simulink model "simluation"  (R2015a)
settings: Solver=ode45  StartTime=0.0  StopTime=10.0  RelTol=1e-3
libraries: simulink x8
settings Model: Creator=Scott  LastModifiedBy=Scott

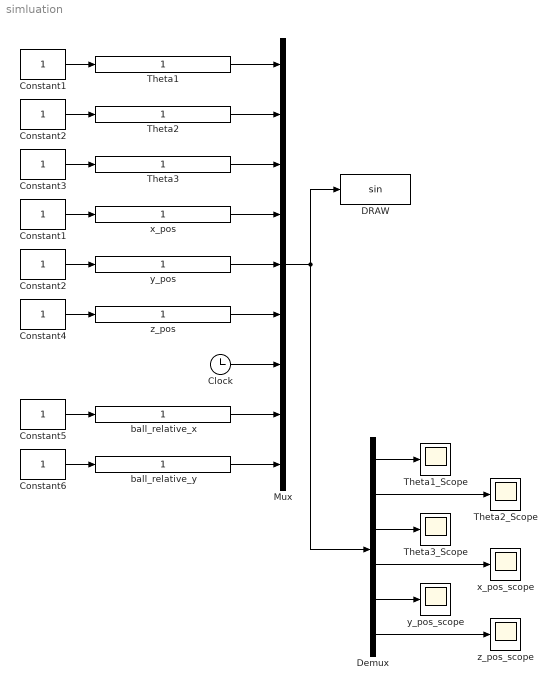
== system simluation ==
  Clock : Clock
  Constant{1..6} (6 alike) : Constant
  "Constant1 " : Constant
  "Constant2 " : Constant
  DRAW : MATLABFcn
  Demux : Demux  Outputs=6
  Mux : Mux  Inputs=9
  Theta1 : simulink/Math Operations/Slider Gain  low=0  gain=1  high=2
  "Theta1_Scope " : Scope
  "Theta2 " : simulink/Math Operations/Slider Gain  low=0  gain=1  high=2
  "Theta2_Scope " : Scope
      settings: SaveName=ScopeData3
  Theta3 : simulink/Math Operations/Slider Gain  low=0  gain=1  high=2
  Theta3_Scope : Scope
  ball_relative_x : simulink/Math Operations/Slider Gain  low=0  gain=1  high=2
  ball_relative_y : simulink/Math Operations/Slider Gain  low=0  gain=1  high=2
  x_pos : simulink/Math Operations/Slider Gain  low=0  gain=1  high=2
  x_pos_scope : Scope
      settings: SaveName=ScopeData4
  y_pos : simulink/Math Operations/Slider Gain  low=0  gain=1  high=2
  y_pos_scope : Scope
      settings: SaveName=ScopeData2
  z_pos : simulink/Math Operations/Slider Gain  low=0  gain=1  high=2
  z_pos_scope : Scope
      settings: SaveName=ScopeData5
  wires:
  Mux/1 -> Demux/1, DRAW/1
  Theta1/1 -> Mux/1
  "Constant1 "/1 -> Theta1/1
  "Theta2 "/1 -> Mux/2
  Theta3/1 -> Mux/3
  "Constant2 "/1 -> "Theta2 "/1
  Constant3/1 -> Theta3/1
  x_pos/1 -> Mux/4
  y_pos/1 -> Mux/5
  z_pos/1 -> Mux/6
  Constant1/1 -> x_pos/1
  Constant2/1 -> y_pos/1
  Constant4/1 -> z_pos/1
  Demux/1 -> "Theta1_Scope "/1
  Demux/2 -> "Theta2_Scope "/1
  Demux/3 -> Theta3_Scope/1
  Demux/4 -> x_pos_scope/1
  Demux/5 -> y_pos_scope/1
  Demux/6 -> z_pos_scope/1
  Clock/1 -> Mux/7
  Constant5/1 -> ball_relative_x/1
  ball_relative_x/1 -> Mux/8
  ball_relative_y/1 -> Mux/9
  Constant6/1 -> ball_relative_y/1
